simulink model "Part2"  (R2018b)
settings: Solver=VariableStepAuto  StartTime=0.0  StopTime=20.0  RelTol=1e-3
settings Model: Creator=Rasouli  LastModifiedBy=Rasouli

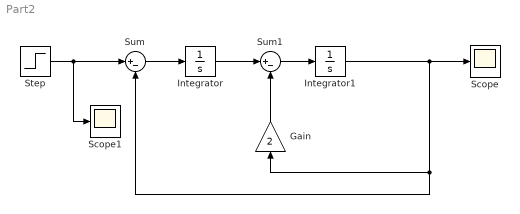
== system Part2 ==
  Gain : Gain  Gain=2
  Integrator : Integrator
  Integrator1 : Integrator
  Scope : Scope
  Scope1 : Scope
  Step : Step  Time=0.001  SampleTime=0
  Sum : Sum  Inputs=|+-
  Sum1 : Sum  Inputs=|+-
  wires:
  Sum1/1 -> Integrator1/1
  Integrator/1 -> Sum1/1
  Step/1 -> Scope1/1, Sum/1
  Sum/1 -> Integrator/1
  Integrator1/1 -> Scope/1, Gain/1, Sum/2
  Gain/1 -> Sum1/2
